simulink model "GUAM"  (R2023b)
settings: Solver=FixedStepAuto  StartTime=0.0  StopTime=SimIn.stopTime  FixedStep=Ts  RelTol=1e-3  AbsTol=1e-4  EnableMultiTasking=on
PostLoadFcn:
  | warning('off','sm:sli:setup:compile:LocalSolverNotSupported')
StartFcn:
  | tic
StopFcn:
  | Elapsed_Sim_Time = toc;
model workspace: external: MATLAB File aileronAssembly_DataFile.m (data not in the file)
values from neighbouring files (symbols this model uses):
  Ts = 0.05    [RUNME.m]
undefined symbols (not defined in the file or in its folder): AAC_Param, ang2Ext_coeff, Ki, Ki_scaling_elec, Kp, Leadscrew, motor_friction, R7_sctrl, sigbuilder_block, SimIn, SimPar, sm_aileron_actuator_lib, smiData, X, Y, Z
libraries: sm_lib x608, fl_lib x378, ee_lib x105, nesl_utility x96, simulink x10, eeGeneralControl x7, sh_lib x7, dspstat3 x6, sdl_lib x3, slpidlib x2, aerolibfltsims x2
(part 1 of 22)
Description:
  | Aileron Actuation System
  | 
  | Copyright 2018-2022 The MathWorks, Inc.
settings Model: NumberOfSteps=4  PacingRate=0.100000  Creator=smiller  LastModifiedBy=mkhaleghi
settings SolverCC: ConcurrentTasks=on  PositivePriorityOrder=on  AutoInsertRateTranBlk=on  InsertRTBMode=Never (minimum delay)
settings DataIOCC: MaxDataPoints=15000  SaveFormat=StructureWithTime  ReturnWorkspaceOutputs=off  SignalLoggingName=logsout_sm_aileron_actuator
settings OptimizationCC: BlockReduction=off  OptimizeBlockIOStorage=off  BufferReuse=off  ReuseModelBlockBuffer=off  GlobalBufferReuse=off  ExpressionFolding=off  LocalBlockOutputs=off  ZeroExternalMemoryAtStartup=off  ZeroInternalMemoryAtStartup=off  OptimizeDataStoreBuffers=off  BusAssignmentInplaceUpdate=off
settings DebuggingCC: UnconnectedInputMsg=warning  UnconnectedOutputMsg=warning  UnconnectedLineMsg=warning  PregeneratedLibrarySubsystemCodeDiagnostic=none  ArithmeticOperatorsInVariantConditions=warning
settings ModelReferenceCC: EnableRefExpFcnMdlSchedulingChecks=on
settings SFSimCC: SimUseLocalCustomCode=off  CustomCodeUndefinedFunction=UseInterfaceOnly
settings RTWCC: RTWUseLocalCustomCode=off  Toolchain=Simulink Real-Time Toolchain  BuildConfiguration=Faster Runs  TargetLang=C++  DLArmComputeVersion=19.05
settings GRTTargetCC: TargetLangStandard=C++03 (ISO)  CodeInterfacePackaging=C++ class
settings SimscapeCC: SimscapeLogType=all  SimscapeLogSimulationStatistics=on  SimscapeLogName=simlog_sm_aileron_actuator  SimscapeLogDataHistory=15000
settings DiagnosticsConfigSet: SimMechanicsJointTargetOverSpecification=none
settings ExplorerConfigSet: InternalSimMechanicsExplorerSettings="<ExplorerConfiguration><canonicalview>default</canonicalview><AnimationSetting><BasePlaybackSpeed>1.0</BasePlaybackSpeed><PlaybackSpeedFactor>1.0</PlaybackSpeedFactor></AnimationSetting><TilePanel><TileInfo><Tiles Columns=\"1\" Count=\"2\" Rows=\"2\"><Column Weight=\"1\"/><Row Weight=\"0.4705\"/><Row Weight=\"0.5295\"/><Tile Height=\"1\" Width=\"1\" X=\"0\" Y=\"0\"/><Tile Height=\"1\" Width=\"1\" X=\"0\" Y=\"1\"/></Tiles></TileInfo><SceneInfo><SceneViewer><BGColor><R>1</R><G>1</G><B>1</B></BGColor><Camera><DoPerspective>off</DoPerspective><Position><X>1.23761627695084986</X><Y>-8.90758678936009929</Y><Z>1.00676905686621598</Z></Position><Center><X>1.32324875041682244</X><Y>-5.82226757680397977</Y><Z>0.958078552790263771</Z></Center><Up><X>0.0220880463597219329</X><Y>0.0151626360058847443</Y><Z>0.999641041913228001</Z></Up><ViewLimDist>1</ViewLimDist><YLim>0.212915807710631483</YLim><XLim>0.504029784798622149</XLim></Camera></SceneViewer><SceneViewer><BGColor><R>1</R><G>1</G><B>1</B></BGColor><Camera><DoPerspective>off</DoPerspective><Position><X>0.794396209708300383</X><Y>-9.38995557415099746</Y><Z>3.30429825173386327</Z></Position><Center><X>1.22507763881924903</X><Y>-6.96050137175265426</Y><Z>-0.946177962255213334</Z></Center><Up><X>0.0136714074370919147</X><Y>0.867510835818079196</Y><Z>0.497230371514961633</Z></Up><ViewLimDist>1</ViewLimDist><YLim>0.0698383925509900721</YLim><XLim>0.146660624357079161</XLim></Camera></SceneViewer></SceneInfo></TilePanel><MechEditorPanel><Cameras/><GfxPanelCameraMap/><VideoCreator><PlaybackSpeedRatio>1.0</PlaybackSpeedRatio><FrameRate>30</FrameRate><VideoFormat>Motion JPEG AVI</VideoFormat><FrameSize>auto</FrameSize></VideoCreator></MechEditorPanel></ExplorerConfiguration>"

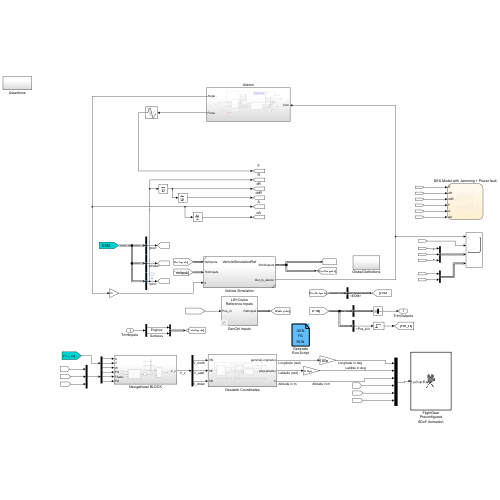
[thumbnail: Simulink's stored preview of the top-level diagram]
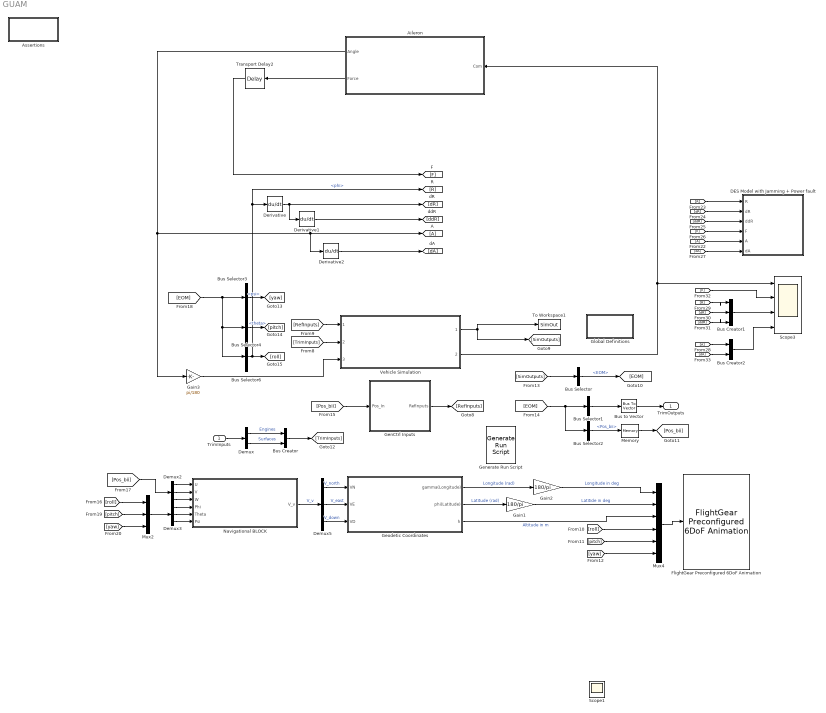
== system GUAM ==
  TrimInputs : Inport
  A : Goto
  Aileron : Subsystem
  Assertions : Subsystem
  Bus Creator : BusCreator  Inputs=2  OutDataTypeStr=Bus: BUS_TRIM_INPUT
  Bus Creator1 : BusCreator  Inputs=3
  Bus Creator2 : BusCreator  Inputs=2
  Bus Selector : BusSelector  OutputSignals=Vehicle.EOM
  Bus Selector1 : BusSelector  OutputSignals=AirRelativeData.Veas,AirRelativeData.Vtot,AirRelativeData.alpha,AirRelativeData.beta,WorldRelativeData.gamma,WorldRelativeData.chi,InertialData.Asensed_bIb,AirRelativeData.Vtotdot,AirRelativeData.alphadot,AirRelativeData.betadot,WorldRelativeData.gammadot,WorldRelativeData.chidot,WorldRelativeData.VelDtH_bEh,WorldRelativeData.Euler.phi,WorldRelativeData.Euler.theta,WorldRelativeData.Euler.psi  OutputAsBus=on
  Bus Selector2 : BusSelector  OutputSignals=InertialData.Pos_bii
  Bus Selector3 : BusSelector  OutputSignals=WorldRelativeData.Euler.psi
  Bus Selector4 : BusSelector  OutputSignals=WorldRelativeData.Euler.theta
  Bus Selector6 : BusSelector  OutputSignals=WorldRelativeData.Euler.phi
  Bus to Vector : BusToVector
  DES Model with Jamming + Power fault : Stateflow chart  TreatAsAtomicUnit=on
      settings: PortSchema="{\"entries\":[{\"content\":{\"sides\":[{\"content\":{},\"type\":\"ConnectorPlacement.EquallySpacedRectSide\",\"uuid\":\"a67ccfb6-3a22-4184-959b-082339053208\"},{\"content\":{\"side\":\"RIGHT\"},\"type\":\"ConnectorPlacement.EquallySpacedRectSide\",\"uuid\":\"6d92a68e-2e9e-4c9c-ac97-2465a38c08e0\"},{\"content\":{\"side\":\"TOP\"},\"type\":\"ConnectorPlacement.EquallySpacedRectSide\",\"uuid\":\"ae8db2dd-ba89-4797-9154-20cef1450f5e\"},{\"content\":{\"connectorIds\":[\"In1\",\"In2\",\"In5\",\"In4\",\"In3\",\"In6\"],\"side\":\"BOTTOM\"},\"type\":\"ConnectorPlacement.EquallySpacedRectSide\",\"uuid\":\"4d772bfb-b5db-457d-b647-bdd980a0fe5b\"}]},\"type\":\"ConnectorPlacement.EquallySpacedConnector\",\"uuid\":\"6e87b71b-43ed-4efe-bae7-cb7d2639d285\"}],\"packageUris\":[\"http://schema.mathworks.com/mf0/Connector/R2020b\"],\"version\":\"1.0\"}"
  Demux : Demux  Outputs=[SimIn.Trim.numEngines SimIn.Trim.numSurfaces]
  Demux2 : Demux  Outputs=3
  Demux3 : Demux  Outputs=3
  Demux5 : Demux  Outputs=3
  Derivative : Derivative
  Derivative1 : Derivative
  Derivative2 : Derivative
  FlightGear Preconfigured 6DoF Animation : aerolibfltsims/FlightGear Preconfigured 6DoF Animation  xFlightGearVersion=v2019.1  DestinationIpAddress=127.0.0.1  DestinationPort=5502  SampleTime=Ts  packetVersion=24
  From22 : From
  From28 : From
  Gain1 : Gain  Gain=180/pi
  Gain2 : Gain  Gain=180/pi
  Gain3 : Gain  Gain=pi/180
  GenCtrl Inputs : Subsystem  Variant=on  VariantControl=Variant1
  Generate Run Script : aerolibfltsims/Generate Run Script  Architecture=Win64  dataFlow=Send  GeometryModelName=c172p  AirportId=KJFK  RunwayId=13L  InitialAltitude=1100  InitialHeading=113  OffsetDistance=0  OffsetAzimuth=0  InstallScenery=off  DisableShaders=on  OriginAddress=127.0.0.1  DestinationPort=5502  OriginPort=5505  LocalAddress=127.0.0.1  OutputFileName=runfg.bat  FlightGearBaseDirectory=C:\Program Files\FlightGear 2020.3
  Geodetic Coordinates : Subsystem
  Global Definitions : Subsystem
  Memory : Memory
  Mux2 : Mux  Inputs=3
  Mux4 : Mux  Inputs=6
  Navigational BLOCK : Subsystem
  Scope3 : Scope  NumInputPorts=4
  To Workspace1 : ToWorkspace  VariableName=SimOut  SaveFormat=Timeseries  SampleTime=-1
      settings: Save2DSignal=2-D array (concatenate along first dimension)
  Transport Delay2 : TransportDelay  DelayTime=0.3
  Vehicle Simulation : Subsystem  ReferencedSubsystem=VehicleSimulationRef
  TrimOutputs : Outport  OutDataTypeStr=double  VectorParamsAs1DForOutWhenUnconnected=off
  Scope1 : Scope
  wires:
  Bus Selector4/1 -> [pitch]  "<theta>"
  [pitch] -> Mux4/5
  [pitch] -> Mux2/2
  Demux3/3 -> Navigational BLOCK/6(Psi)
  Gain1/1 -> Mux4/2  "Latitide in deg"
  [Pos_bii] -> GenCtrl Inputs/1(Pos_In)
  Mux2/1 -> Demux3/1
  Demux3/2 -> Navigational BLOCK/5(Theta)
  Geodetic Coordinates/3(h) -> Mux4/3  "Altitude in m"
  Geodetic Coordinates/1(gamma(Longitude)) -> Gain2/1  "Longitude (rad)"
  Bus Selector3/1 -> [yaw]  "<psi>"
  Bus Selector1/1 -> Bus to Vector/1
  Demux5/1 -> Geodetic Coordinates/1(VN)  "V_north"
  Demux5/3 -> Geodetic Coordinates/3(VD)  "V_down"
  Geodetic Coordinates/2(phi(Latitude)) -> Gain1/1  "Latitude (rad)"
  Demux2/2 -> Navigational BLOCK/2(V)
  [EOM] -> Bus Selector6/1, Bus Selector4/1, Bus Selector3/1
  [yaw] -> Mux2/3
  Navigational BLOCK/1(V_v) -> Demux5/1  "V_v"
  Demux2/1 -> Navigational BLOCK/1(U)
  [EOM] -> Bus Selector1/1, Bus Selector2/1
  Demux3/1 -> Navigational BLOCK/4(Phi)
  Bus Selector/1 -> [EOM]  "<EOM>"
  Memory/1 -> [Pos_bii]
  Demux2/3 -> Navigational BLOCK/3(W)
  GenCtrl Inputs/1(RefInputs) -> [RefInputs]
  [roll] -> Mux4/4
  Bus Selector2/1 -> Memory/1  "<Pos_bii>"
  Demux5/2 -> Geodetic Coordinates/2(VE)  "V_east"
  [RefInputs] -> Vehicle Simulation/1
  [yaw] -> Mux4/6
  Vehicle Simulation/1 -> To Workspace1/1, [SimOutputs]
  [roll] -> Mux2/1
  [TrimInputs] -> Vehicle Simulation/2
  Demux/1 -> Bus Creator/1  "Engines"
  [SimOutputs] -> Bus Selector/1
  TrimInputs/1 -> Demux/1
  Mux4/1 -> FlightGear Preconfigured 6DoF Animation/1
  Bus to Vector/1 -> TrimOutputs/1
  Bus Selector6/1 -> [roll], [R], Derivative/1  "<phi>"
  Gain2/1 -> Mux4/1  "Longitude in deg"
  Bus Creator/1 -> [TrimInputs]
  [Pos_bii] -> Demux2/1
  Demux/2 -> Bus Creator/2  "Surfaces"
  Gain3/1 -> Vehicle Simulation/3
  Vehicle Simulation/2 -> Scope3/1, Aileron/1(Com)
  Derivative/1 -> [dR], Derivative1/1
  Derivative1/1 -> [ddR]
  Aileron/1(Angle) -> Gain3/1, Derivative2/1, A/1
  Aileron/2(Force) -> Transport Delay2/1
  Transport Delay2/1 -> [F]
  Derivative2/1 -> [dA]
  [R] -> DES Model with Jamming + Power fault/1(R)
  [dR] -> DES Model with Jamming + Power fault/2(dR)
  [ddR] -> DES Model with Jamming + Power fault/5(ddR)
  [F] -> DES Model with Jamming + Power fault/4(F)
  From22/1 -> DES Model with Jamming + Power fault/3(A)
  [dA] -> DES Model with Jamming + Power fault/6(dA)
  [F] -> Scope3/2
  [R] -> Bus Creator1/1
  [dR] -> Bus Creator1/2
  [ddR] -> Bus Creator1/3
  Bus Creator1/1 -> Scope3/3
  From28/1 -> Bus Creator2/1
  [dA] -> Bus Creator2/2
  Bus Creator2/1 -> Scope3/4

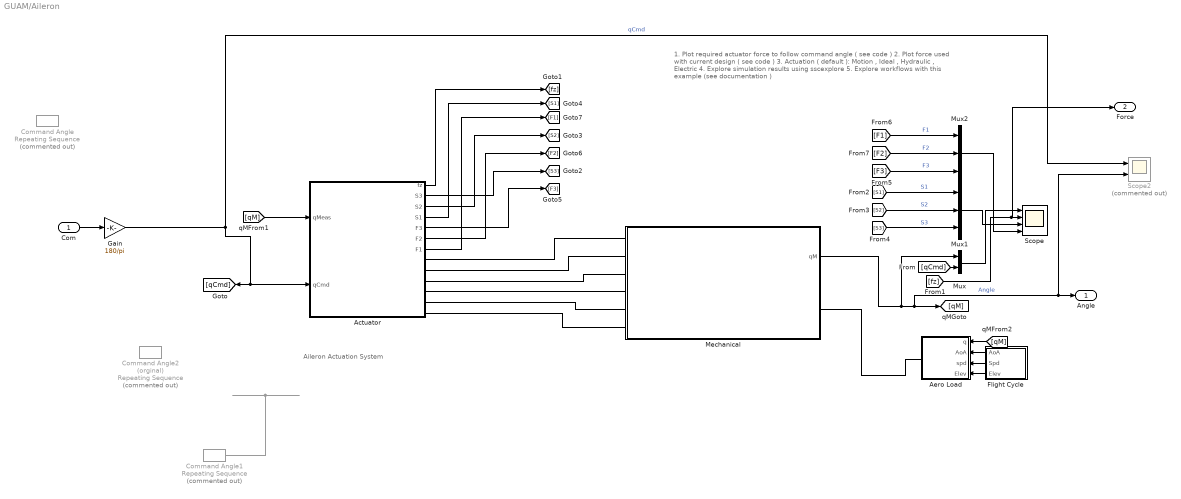
== system GUAM/Aileron ==
  note: 1. Plot required actuator force to follow command angle ( see code )
      | 2. Plot force used with current design ( see code )
      | 3. Actuation ( default ): Motion , Ideal , Hydraulic , Electric
      | 4. Explore simulation results using sscexplore
      | 5. Explore workflows with this example (see documentation )
  note: Aileron Actuation System
  Com : Inport
  Actuator : Subsystem  Tag=PublishSubsystem  Variant=on  VariantControlMode=label  VariantControl=Variant1  LabelModeActiveChoice=Electric
      settings: AttributesFormatString=%<ActiveVariant>
      mask Display:
      | Act_Char = get_param([bdroot '/Actuator'],'ActiveVariant');
      | SnC_Char = 'X';
      | PWM_Char = 'X';
      | if(strcmp(Act_Char(1),'E'))
      |     SnC_Char = get_param([bdroot '/Actuator/Electric/Leadscrew 1'],'popup_ctrl');
      |     PWM_Char = get_param([bdroot '/Actuator/Electric/Leadscrew 1'],'popup_driver');
      | end
      | 
      | image_str = ['sm_aileron_actuator_' Act_Char(1) 'sc' upper(SnC_Char(1)) 'pw' PWM_Char(1) '_IMAGE.png'];
      | 
      | try
      |     image(image_str);
      | catch
      | 
      | end
  Aero Load : Subsystem
  Command Angle : simulink/Sources/Repeating Sequence  Commented=on  rep_seq_t="[0.0 0.5 1.0 1.5  2.0  2.5  3.0   3.5  4.0   4.5    5.0   5.5  6.0   6.5  7.0   7.5  8.0  8.5  9.0  9.5   10.0]"  rep_seq_y="[0.0  0.0  0.0  0.0 5.0  10.0  10.0  0.0  0.0  -9.0  -17.5  -17.5  -10.0  0.0  2.0  6.0 15.0 15.0 6.0 3.0 -2.0]"
  Command Angle1 : simulink/Sources/Repeating Sequence  Commented=on  rep_seq_t="[0.0 0.5 1.0 1.5  2.0  2.5  3.0   3.5  4.0   4.5    5.0   5.5  6.0   6.5  7.0   7.5  8.0  8.5  9.0  9.5   10.0 10.5 11.0 11.5 12.0 12.5 13.0]"  rep_seq_y=|
      | [0
      | 0
      | 0
      | 0
      | 5
      | 10
      | 10
      | 0
      | 0
      | -10
      | -10
      | -10
      | 0
      | 0
      | 0
      | 6
      | 15
      | 15
      | 6
      | 0
      | -5
      | -5
      | 0
      | 0
      | 5
      | 10
      | 10]
  Command Angle2 (orginal) : simulink/Sources/Repeating Sequence  Commented=on  rep_seq_t="[0.0 0.5 1.0 1.5  2.0  2.5  3.0   3.5  4.0   4.5    5.0   5.5  6.0   6.5  7.0   7.5  8.0  8.5  9.0  9.5   10.0 10.5 11.0 11.5 12.0 12.5 13.0]"  rep_seq_y="[0.0  0.0  0.0  0.0 5.0  10.0  10.0  0.0  0.0  -9.0  -17.5  -17.5  -10.0  0.0  2.0  6.0 15.0 15.0 6.0 3.0 -2.0 -2.0 0 3.0 5.0 6.0 6.0]"
  Flight Cycle : Subsystem  Tag=STV Subsys  LoadFcn=sigbuilder_block('load');  StartFcn=sigbuilder_block('start');  StopFcn=sigbuilder_block('stop');  ClipboardFcn=sigbuilder_block('clipboard');  mask(Sigbuilder block){tuvar=[0:10]}
      mask help: Simulink:masks:SigbuilderBlock_MD
      mask init:
      | if ~strcmp(get_param(bdroot(gcbh),'SimulationStatus'),'stopped') tuvar = sigbuilder_block('maskInit'); end
      settings: CopyFcn=sigbuilder_block('copy');  DeleteFcn=sigbuilder_block('delete');  ModelCloseFcn=sigbuilder_block('modelClose');  PreSaveFcn=sigbuilder_block('preSave');  PauseFcn=sigbuilder_block('pause');  ContinueFcn=sigbuilder_block('continue');  NameChangeFcn=sigbuilder_block('namechange');  OpenFcn=sigbuilder_block('open',[440.4 133.2 550.8 400.2 ]);  CloseFcn=sigbuilder_block('close');
      mask Display: plot(0, 0, 100, 100,[2, 2, 32, 32, 2], [68, 8, 8, 68, 68],[32, 2], [38, 38], [32, 19, 2],[53, 60, 44], [32, 17, 17, 2],[16, 16, 31, 31]);txt = getActiveGroup(gcbh);text(2, 100, txt,'verticalAlignment', 'top');
  Gain : Gain  Gain=180/pi
  Mechanical : Subsystem  Tag=PublishSubsystem
      mask Display: image('sm_aileron_actuator_aileron_full_IMAGE.png');
  Mux : Mux  Inputs=2
  Mux1 : Mux  Inputs=3
  Mux2 : Mux  Inputs=3
  Scope : Scope  NumInputPorts=4
  Scope2 : Scope  Commented=on  NumInputPorts=2
  Angle : Outport
  Force : Outport  Port=2
  wires:
  Command Angle1/1 -> ?
  Mux1/1 -> Scope/3
  Mux/1 -> Scope/1
  Mux2/1 -> Scope/4
  [F3] -> Mux2/3  "F3"
  Actuator/3(S2) -> [S2]
  Gain/1 -> Scope2/1, Actuator/2("qCmd "), [qCmd]  "qCmd"
  Actuator/4(S1) -> [S1]
  Actuator/6(F2) -> [F2]
  Flight Cycle/2(Spd) -> Aero Load/3(spd)
  Actuator/5(F3) -> [F3]
  [F2] -> Mux2/2  "F2"
  Actuator/7(F1) -> [F1]
  [qM] -> Aero Load/1(q)
  Flight Cycle/3(Elev) -> Aero Load/4(Elev)
  [qM] -> Actuator/1(qMeas)
  Actuator/2(S3) -> [S3]
  Mechanical/1(qM) -> Angle/1, Scope2/2, [qM], Mux/1  "Angle"
  [S1] -> Mux1/1  "S1"
  [fz] -> Force/1, Scope/2
  [S3] -> Mux1/3  "S3"
  [qCmd] -> Mux/2
  [F1] -> Mux2/1  "F1"
  Flight Cycle/1(AoA) -> Aero Load/2(AoA)
  Actuator/1(" fz") -> [fz]
  [S2] -> Mux1/2  "S2"
  Com/1 -> Gain/1
  connections:
  Actuator/RConn3 -- Mechanical/LConn3
  Actuator/RConn4 -- Mechanical/LConn4
  Actuator/RConn5 -- Mechanical/LConn5
  Aero Load/RConn1 -- Mechanical/RConn1
  Actuator/RConn6 -- Mechanical/LConn6
  Actuator/RConn1 -- Mechanical/LConn1
  Actuator/RConn2 -- Mechanical/LConn2

== system GUAM/Assertions ==
  Clock1 : Clock
  Compare To Constant : simulink/Logic and Bit Operations/Compare To Constant  relop=>=  const=0.2  OutDataTypeStr=boolean  ZeroCross=off
  Constant2 : Constant  Value=SimIn.Switches.TrimModeOn
  Constant3 : Constant  Value=SimIn.Switches.LinearizeModeOn
  KillifNotSimMode : Assertion  AssertionFailFcn="warndlg('Running simulation with TrimMode or LinearizeMode engaged.  Run setup.m to reset.','Warning!')"
  Logical Operator : Logic  Operator=NAND  AllPortsSameDT=off  OutDataTypeStr=boolean
  Logical Operator1 : Logic  Operator=OR  AllPortsSameDT=off  OutDataTypeStr=boolean
  wires:
  Constant2/1 -> Logical Operator1/1
  Compare To Constant/1 -> Logical Operator/2
  Clock1/1 -> Compare To Constant/1
  Logical Operator/1 -> KillifNotSimMode/1
  Constant3/1 -> Logical Operator1/2
  Logical Operator1/1 -> Logical Operator/1

== system GUAM/GenCtrl Inputs ==
  Pos_In : Inport
  GL-10 Reference Inputs : Subsystem  VariantControl=GVS_VEH_TYPE_GL10  ReferencedSubsystem=GL_10_Reference_Inputs
  Generic Tilt Rotor Reference Inputs : Subsystem  VariantControl=GVS_VEH_TYPE_GTR  ReferencedSubsystem=GTR_Reference_Inputs
  Generic Tilt Wing Reference Inputs : Subsystem  VariantControl=GVS_VEH_TYPE_GTW  ReferencedSubsystem=GTW_Reference_Inputs
  LA-8 Reference Inputs : Subsystem  VariantControl=GVS_VEH_TYPE_LA8  ReferencedSubsystem=LA_8_Reference_Inputs
  Lift+Cruise Reference Inputs : Subsystem  VariantControl=GVS_VEH_TYPE_LC  ReferencedSubsystem=Lift_Cruise_Reference_Inputs
  Quad6 Reference Inputs : Subsystem  VariantControl=GVS_VEH_TYPE_QUAD6  ReferencedSubsystem=Quad6_Reference_Inputs
  RefInputs : Outport  OutDataTypeStr=Bus: BUS_REF_INPUT

== system GUAM/Geodetic Coordinates ==
  VN : Inport
  VE : Inport  Port=2
  VD : Inport  Port=3
  Gain : Gain  Gain=-1
  Integrator : Integrator  InitialCondition=150
  Integrator1 : Integrator  InitialCondition=0.22181
  Integrator2 : Integrator  InitialCondition=1.356068
  LATITUDE : MATLAB Function  TreatAsAtomicUnit=on
  LONGITUDE : MATLAB Function  TreatAsAtomicUnit=on
  M and N : Subsystem
  gamma(Longitude) : Outport
  phi(Latitude) : Outport  Port=2
  h : Outport  Port=3
  wires:
  VD/1 -> Gain/1  "VD"
  Gain/1 -> Integrator/1  "h_dot"
  Integrator/1 -> LATITUDE/3(h), LONGITUDE/3(h), h/1  "h"
  M and N/1(M) -> LATITUDE/2(M)
  M and N/2(N) -> LONGITUDE/2(N)
  LATITUDE/1(phi_dot) -> Integrator1/1  "phi_dot"
  Integrator1/1 -> LONGITUDE/4(phi), M and N/1(phi), phi(Latitude)/1  "phi"
  VE/1 -> LONGITUDE/1(VE)  "VE"
  VN/1 -> LATITUDE/1(VN)  "VN"
  LONGITUDE/1(gamma_dot) -> Integrator2/1  "gamma_dot"
  Integrator2/1 -> gamma(Longitude)/1  "gamma"

== system GUAM/Global Definitions ==
  EOM_IC : Constant  Value=SimPar.EOM  OutDataTypeStr=Bus: BUS_PARAM_EOM
  IC : Constant  Value=SimPar.IC  OutDataTypeStr=Bus: BUS_PARAM_IC
  Terminator : Terminator
  Terminator1 : Terminator
  tag scope: EOM_IC=global, IC=global
  wires:
  IC/1 -> [IC]
  EOM_IC/1 -> [EOM_IC]
  [IC] -> Terminator/1
  [EOM_IC] -> Terminator1/1

== system GUAM/Navigational BLOCK ==
  U : Inport
  V : Inport  Port=2
  W : Inport  Port=3
  Phi : Inport  Port=4
  Theta : Inport  Port=5
  Psi : Inport  Port=6
  Math Function : Math  Operator=transpose
  Matrix Multiply : Product  Multiplication=Matrix(*)
  Mux2 : Mux  Inputs=3
  Navigational Equation : Subsystem
  V_v : Outport
  wires:
  V/1 -> Mux2/2
  Psi/1 -> Navigational Equation/3(phi)
  W/1 -> Mux2/3
  Navigational Equation/1(C_B/V) -> Math Function/1
  Matrix Multiply/1 -> V_v/1
  Theta/1 -> Navigational Equation/2(theat)
  U/1 -> Mux2/1
  Phi/1 -> Navigational Equation/1(psi)
  Math Function/1 -> Matrix Multiply/1
  Mux2/1 -> Matrix Multiply/2

== system GUAM/Aileron/Actuator ==
  qMeas : Inport
  "qCmd " : Inport  Port=2
  Electric : Subsystem  VariantControl=Electric
      mask Display: image('sm_aileron_actuator_EscXpwX_IMAGE.png');
  Hydraulic : Subsystem  VariantControl=Hydraulic
      mask Display: image('sm_aileron_actuator_HscXpwX_IMAGE.png');
  Ideal : Subsystem  VariantControl=Ideal
      mask Display: image('sm_aileron_actuator_IscXpwX_IMAGE.png');
  Motion : Subsystem  VariantControl=Motion
      mask Display: image('sm_aileron_actuator_MscXpwX_IMAGE.png');
  " C1" : PMIOPort  Side=Right
  " P1" : PMIOPort  Port=2  Side=Right
  " C2" : PMIOPort  Port=3  Side=Right
  " P2" : PMIOPort  Port=4  Side=Right
  " C3" : PMIOPort  Port=5  Side=Right
  " P3" : PMIOPort  Port=6  Side=Right
  " fz" : Outport  VectorParamsAs1DForOutWhenUnconnected=off
  S3 : Outport  Port=2
  S2 : Outport  Port=3
  S1 : Outport  Port=4
  F3 : Outport  Port=5
  F2 : Outport  Port=6
  F1 : Outport  Port=7

== system GUAM/Aileron/Aero Load ==
  note: Proof of concept calculation only.
      | Realistic values must be obtained from literature or experimentation.
  q : Inport
  AoA : Inport  Port=2
  spd : Inport  Port=3
  Elev : Inport  Port=4
  Aerodynamic Hinge Moment : sm_lib/Forces and Torques/External Force and Torque  ForceResolutionFrame=AttachedFrame  EnableForceX=off  EnableForceY=off  EnableForceZ=off  EnableForce=off  TorqueResolutionFrame=AttachedFrame  EnableTorqueX=off  EnableTorqueY=on  EnableTorqueZ=off  EnableTorque=off
  Gain : Gain  Gain=0.5
  Math Function : Math  Operator=square  SignedPower=on
  Product : Product  Inputs=4
  Scaling : Gain  Gain=1e-6
  Simulink-PS Converter : nesl_utility/Simulink-PS Converter  PhysicalDomain=network_engine_domain  SubClassName=ps_input  LeftPortType=input  RightPortType=output  PseudoPeriodic=off  Frequencies=[]  NoiseDistribution=none  NoiseParameters=[]  Unit=1  AffineConversion=off  FilteringAndDerivatives=provide  SimscapeFilterOrder=1  InputFilterTimeConstant=0.005  UdotUserProvided=0
  Table AoA : Lookup_n-D  NumberOfTableDimensions=1  BreakpointsForDimension1=[-5:5]  Table=tanh([-5:5])  InternalRulePriority=Speed  RndMeth=Simplest
  Table Elev : Lookup_n-D  NumberOfTableDimensions=1  BreakpointsForDimension1=[-5:5]  Table=tanh([-5:5])  InternalRulePriority=Speed  RndMeth=Simplest
  Table q : Lookup_n-D  NumberOfTableDimensions=1  BreakpointsForDimension1=[-5:5]  Table=tanh([-5:5])  InternalRulePriority=Speed  RndMeth=Simplest
  A : PMIOPort  Side=Right
  wires:
  Gain/1 -> Scaling/1
  AoA/1 -> Table AoA/1
  q/1 -> Table q/1
  spd/1 -> Math Function/1
  Elev/1 -> Table Elev/1
  Table q/1 -> Product/1
  Table AoA/1 -> Product/2
  Math Function/1 -> Product/3
  Table Elev/1 -> Product/4  "rho"
  Product/1 -> Gain/1
  Scaling/1 -> Simulink-PS Converter/1
  connections:
  Simulink-PS Converter/RConn1 -- Aerodynamic Hinge Moment/LConn1
  Aerodynamic Hinge Moment/RConn1 -- A/RConn1

== system GUAM/Aileron/Flight Cycle ==
  Demux : Demux  Tag=STV Demux  Outputs=3
      settings: DisplayOption=none
  FromWs : FromWorkspace  Tag=STV FromWs  VariableName=tuvar
      SigBuilderData=|
      | common.afterFinalStr = 'Extrapolate'
      | common.sampleTime = 0
      | dataSet.timeRange = [0 10]
      | dataSet.name = 'FC1'
      | sbobj.Groups.Name = 'FC1'
      | sbobj.Groups.Signals(1).Name = 'AoA'
      | sbobj.Groups.Signals(1).XData = [0 10]
      | sbobj.Groups.Signals(1).YData = [1 1]
      | sbobj.Groups.Signals(2).Name = 'Spd'
      | sbobj.Groups.Signals(2).XData = [0 10]
      | sbobj.Groups.Signals(2).YData = [1000 1000]
      | sbobj.Groups.Signals(3).Name = 'Elev'
      | sbobj.Groups.Signals(3).XData = [0 10]
      | sbobj.Groups.Signals(3).YData = [300 300]
  AoA : Outport  Tag=STV Outport  VectorParamsAs1DForOutWhenUnconnected=off
  Spd : Outport  Tag=STV Outport  Port=2  VectorParamsAs1DForOutWhenUnconnected=off
  Elev : Outport  Tag=STV Outport  Port=3  VectorParamsAs1DForOutWhenUnconnected=off
  wires:
  Demux/1 -> AoA/1
  FromWs/1 -> Demux/1
  Demux/2 -> Spd/1
  Demux/3 -> Elev/1

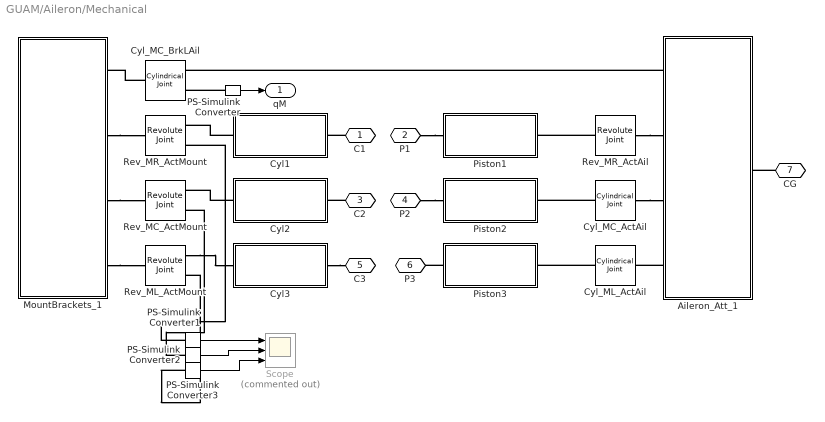
== system GUAM/Aileron/Mechanical ==
  Aileron_Att_1 : Subsystem  Tag=PublishSubsystem
      mask Display: image('sm_aileron_actuator_aileron_assy_IMAGE.png');
  Cyl1 : Subsystem
      mask Display: image('sm_aileron_actuator_aileron_cylinder_IMAGE.png');
  Cyl2 : Subsystem
      mask Display: image('sm_aileron_actuator_aileron_cylinder_IMAGE.png');
  Cyl3 : Subsystem
      mask Display: image('sm_aileron_actuator_aileron_cylinder_IMAGE.png');
  Cyl_MC_ActAil : sm_lib/Joints/Cylindrical Joint  JointMode=Normal  SenseConstraintForce=off  SenseConstraintForceX=off  SenseConstraintForceY=off  SenseConstraintForceZ=off  SenseConstraintTorque=off  SenseConstraintTorqueX=off  SenseConstraintTorqueY=off  SenseConstraintTorqueZ=off  SenseTotalForce=off  SenseTotalForceX=off  SenseTotalForceY=off  SenseTotalForceZ=off  SenseTotalTorque=off  SenseTotalTorqueX=off  SenseTotalTorqueY=off  SenseTotalTorqueZ=off  CompositeWrenchDir=FollowerOnBase  CompositeWrenchFrame=BaseFrame  PzEquilibriumPosition=0  PzEquilibriumPositionUnits=m  PzSpringStiffness=0  PzSpringStiffnessUnits=N/m  PzDampingCoefficient=0  PzDampingCoefficientUnits=N/(m/s)  PzTorqueActuationMode=NoTorque  PzMotionActuationMode=ComputedMotion  PzSensePosition=off  PzSenseVelocity=off  PzSenseAcceleration=off  PzSenseTorqueForce=off  PzSenseLowerLimitTorqueForce=off  PzSenseUpperLimitTorqueForce=off  PzLowerLimitSpecify=off  PzLowerLimitBound=-1  PzLowerLimitBoundUnits=m  PzLowerLimitStiffness=1e6  PzLowerLimitStiffnessUnits=N/m  PzLowerLimitDamping=1e3  PzLowerLimitDampingUnits=N/(m/s)  PzLowerLimitTransitionRegionWidth=1e-4  PzLowerLimitTransitionRegionWidthUnits=m  PzUpperLimitSpecify=off  PzUpperLimitBound=1  PzUpperLimitBoundUnits=m  PzUpperLimitStiffness=1e6  PzUpperLimitStiffnessUnits=N/m  PzUpperLimitDamping=1e3  PzUpperLimitDampingUnits=N/(m/s)  PzUpperLimitTransitionRegionWidth=1e-4  PzUpperLimitTransitionRegionWidthUnits=m  PzPositionTargetSpecify=on  PzPositionTargetPriority=Low  PzPositionTargetValue=smiData.CylindricalJoint(5).Pz.Pos  PzPositionTargetValueUnits=m  PzVelocityTargetSpecify=off  PzVelocityTargetPriority=High  PzVelocityTargetValue=0  PzVelocityTargetValueUnits=m/s  RzEquilibriumPosition=0  RzEquilibriumPositionUnits=rad  RzSpringStiffness=0  RzSpringStiffnessUnits=N*m/rad  RzDampingCoefficient=0  RzDampingCoefficientUnits=N*m/(rad/s)  RzTorqueActuationMode=NoTorque  RzMotionActuationMode=ComputedMotion  RzSensePosition=off  RzSenseVelocity=off  RzSenseAcceleration=off  RzSenseTorqueForce=off  RzSenseLowerLimitTorqueForce=off  RzSenseUpperLimitTorqueForce=off  RzLowerLimitSpecify=off  RzLowerLimitBound=-90  RzLowerLimitBoundUnits=deg  RzLowerLimitStiffness=1e4  RzLowerLimitStiffnessUnits=N*m/deg  RzLowerLimitDamping=10  RzLowerLimitDampingUnits=N*m/(deg/s)  RzLowerLimitTransitionRegionWidth=0.1  RzLowerLimitTransitionRegionWidthUnits=deg  RzUpperLimitSpecify=off  RzUpperLimitBound=90  RzUpperLimitBoundUnits=deg  RzUpperLimitStiffness=1e4  RzUpperLimitStiffnessUnits=N*m/deg  RzUpperLimitDamping=10  RzUpperLimitDampingUnits=N*m/(deg/s)  RzUpperLimitTransitionRegionWidth=0.1  RzUpperLimitTransitionRegionWidthUnits=deg  RzPositionTargetSpecify=on  RzPositionTargetPriority=Low  RzPositionTargetValue=smiData.CylindricalJoint(5).Rz.Pos  RzPositionTargetValueUnits=deg  RzVelocityTargetSpecify=off  RzVelocityTargetPriority=High  RzVelocityTargetValue=0  RzVelocityTargetValueUnits=deg/s
  Cyl_MC_BrkLAil : sm_lib/Joints/Cylindrical Joint  JointMode=Normal  SenseConstraintForce=off  SenseConstraintForceX=off  SenseConstraintForceY=off  SenseConstraintForceZ=off  SenseConstraintTorque=off  SenseConstraintTorqueX=off  SenseConstraintTorqueY=off  SenseConstraintTorqueZ=off  SenseTotalForce=off  SenseTotalForceX=off  SenseTotalForceY=off  SenseTotalForceZ=off  SenseTotalTorque=off  SenseTotalTorqueX=off  SenseTotalTorqueY=off  SenseTotalTorqueZ=off  CompositeWrenchDir=FollowerOnBase  CompositeWrenchFrame=BaseFrame  PzEquilibriumPosition=0  PzEquilibriumPositionUnits=m  PzSpringStiffness=0  PzSpringStiffnessUnits=N/m  PzDampingCoefficient=0  PzDampingCoefficientUnits=N/(m/s)  PzTorqueActuationMode=NoTorque  PzMotionActuationMode=ComputedMotion  PzSensePosition=off  PzSenseVelocity=off  PzSenseAcceleration=off  PzSenseTorqueForce=off  PzSenseLowerLimitTorqueForce=off  PzSenseUpperLimitTorqueForce=off  PzLowerLimitSpecify=off  PzLowerLimitBound=-1  PzLowerLimitBoundUnits=m  PzLowerLimitStiffness=1e6  PzLowerLimitStiffnessUnits=N/m  PzLowerLimitDamping=1e3  PzLowerLimitDampingUnits=N/(m/s)  PzLowerLimitTransitionRegionWidth=1e-4  PzLowerLimitTransitionRegionWidthUnits=m  PzUpperLimitSpecify=off  PzUpperLimitBound=1  PzUpperLimitBoundUnits=m  PzUpperLimitStiffness=1e6  PzUpperLimitStiffnessUnits=N/m  PzUpperLimitDamping=1e3  PzUpperLimitDampingUnits=N/(m/s)  PzUpperLimitTransitionRegionWidth=1e-4  PzUpperLimitTransitionRegionWidthUnits=m  PzPositionTargetSpecify=on  PzPositionTargetPriority=Low  PzPositionTargetValue=smiData.CylindricalJoint(4).Pz.Pos  PzPositionTargetValueUnits=m  PzVelocityTargetSpecify=off  PzVelocityTargetPriority=High  PzVelocityTargetValue=0  PzVelocityTargetValueUnits=m/s  RzEquilibriumPosition=0  RzEquilibriumPositionUnits=rad  RzSpringStiffness=0  RzSpringStiffnessUnits=N*m/rad  RzDampingCoefficient=0  RzDampingCoefficientUnits=N*m/(rad/s)  RzTorqueActuationMode=NoTorque  RzMotionActuationMode=ComputedMotion  RzSensePosition=on  RzSenseVelocity=off  RzSenseAcceleration=off  RzSenseTorqueForce=off  RzSenseLowerLimitTorqueForce=off  RzSenseUpperLimitTorqueForce=off  RzLowerLimitSpecify=off  RzLowerLimitBound=-90  RzLowerLimitBoundUnits=deg  RzLowerLimitStiffness=1e4  RzLowerLimitStiffnessUnits=N*m/deg  RzLowerLimitDamping=10  RzLowerLimitDampingUnits=N*m/(deg/s)  RzLowerLimitTransitionRegionWidth=0.1  RzLowerLimitTransitionRegionWidthUnits=deg  RzUpperLimitSpecify=off  RzUpperLimitBound=90  RzUpperLimitBoundUnits=deg  RzUpperLimitStiffness=1e4  RzUpperLimitStiffnessUnits=N*m/deg  RzUpperLimitDamping=10  RzUpperLimitDampingUnits=N*m/(deg/s)  RzUpperLimitTransitionRegionWidth=0.1  RzUpperLimitTransitionRegionWidthUnits=deg  RzPositionTargetSpecify=on  RzPositionTargetPriority=Low  RzPositionTargetValue=smiData.CylindricalJoint(4).Rz.Pos  RzPositionTargetValueUnits=deg  RzVelocityTargetSpecify=off  RzVelocityTargetPriority=High  RzVelocityTargetValue=0  RzVelocityTargetValueUnits=deg/s
  Cyl_ML_ActAil : sm_lib/Joints/Cylindrical Joint  JointMode=Normal  SenseConstraintForce=off  SenseConstraintForceX=off  SenseConstraintForceY=off  SenseConstraintForceZ=off  SenseConstraintTorque=off  SenseConstraintTorqueX=off  SenseConstraintTorqueY=off  SenseConstraintTorqueZ=off  SenseTotalForce=off  SenseTotalForceX=off  SenseTotalForceY=off  SenseTotalForceZ=off  SenseTotalTorque=off  SenseTotalTorqueX=off  SenseTotalTorqueY=off  SenseTotalTorqueZ=off  CompositeWrenchDir=FollowerOnBase  CompositeWrenchFrame=BaseFrame  PzEquilibriumPosition=0  PzEquilibriumPositionUnits=m  PzSpringStiffness=0  PzSpringStiffnessUnits=N/m  PzDampingCoefficient=0  PzDampingCoefficientUnits=N/(m/s)  PzTorqueActuationMode=NoTorque  PzMotionActuationMode=ComputedMotion  PzSensePosition=off  PzSenseVelocity=off  PzSenseAcceleration=off  PzSenseTorqueForce=off  PzSenseLowerLimitTorqueForce=off  PzSenseUpperLimitTorqueForce=off  PzLowerLimitSpecify=off  PzLowerLimitBound=-0.001  PzLowerLimitBoundUnits=m  PzLowerLimitStiffness=1e6  PzLowerLimitStiffnessUnits=N/m  PzLowerLimitDamping=1e3  PzLowerLimitDampingUnits=N/(m/s)  PzLowerLimitTransitionRegionWidth=1e-4  PzLowerLimitTransitionRegionWidthUnits=m  PzUpperLimitSpecify=off  PzUpperLimitBound=0.001  PzUpperLimitBoundUnits=m  PzUpperLimitStiffness=1e6  PzUpperLimitStiffnessUnits=N/m  PzUpperLimitDamping=1e3  PzUpperLimitDampingUnits=N/(m/s)  PzUpperLimitTransitionRegionWidth=1e-4  PzUpperLimitTransitionRegionWidthUnits=m  PzPositionTargetSpecify=on  PzPositionTargetPriority=Low  PzPositionTargetValue=smiData.CylindricalJoint(6).Pz.Pos  PzPositionTargetValueUnits=m  PzVelocityTargetSpecify=off  PzVelocityTargetPriority=High  PzVelocityTargetValue=0  PzVelocityTargetValueUnits=m/s  RzEquilibriumPosition=0  RzEquilibriumPositionUnits=rad  RzSpringStiffness=0  RzSpringStiffnessUnits=N*m/rad  RzDampingCoefficient=0  RzDampingCoefficientUnits=N*m/(rad/s)  RzTorqueActuationMode=NoTorque  RzMotionActuationMode=ComputedMotion  RzSensePosition=off  RzSenseVelocity=off  RzSenseAcceleration=off  RzSenseTorqueForce=off  RzSenseLowerLimitTorqueForce=off  RzSenseUpperLimitTorqueForce=off  RzLowerLimitSpecify=off  RzLowerLimitBound=-90  RzLowerLimitBoundUnits=deg  RzLowerLimitStiffness=1e4  RzLowerLimitStiffnessUnits=N*m/deg  RzLowerLimitDamping=10  RzLowerLimitDampingUnits=N*m/(deg/s)  RzLowerLimitTransitionRegionWidth=0.1  RzLowerLimitTransitionRegionWidthUnits=deg  RzUpperLimitSpecify=off  RzUpperLimitBound=90  RzUpperLimitBoundUnits=deg  RzUpperLimitStiffness=1e4  RzUpperLimitStiffnessUnits=N*m/deg  RzUpperLimitDamping=10  RzUpperLimitDampingUnits=N*m/(deg/s)  RzUpperLimitTransitionRegionWidth=0.1  RzUpperLimitTransitionRegionWidthUnits=deg  RzPositionTargetSpecify=on  RzPositionTargetPriority=Low  RzPositionTargetValue=smiData.CylindricalJoint(6).Rz.Pos  RzPositionTargetValueUnits=deg  RzVelocityTargetSpecify=off  RzVelocityTargetPriority=High  RzVelocityTargetValue=0  RzVelocityTargetValueUnits=deg/s
  MountBrackets_1 : Subsystem
      mask Display: image('sm_aileron_actuator_aileron_mounts_all_IMAGE.png');
  PS-Simulink Converter : nesl_utility/PS-Simulink Converter  PhysicalDomain=network_engine_domain  SubClassName=ps_output  LeftPortType=input  RightPortType=output  PseudoPeriodic=off  Frequencies=[]  VectorFormat=1-D array  Unit=deg  AffineConversion=off
  PS-Simulink Converter1 : nesl_utility/PS-Simulink Converter  PhysicalDomain=network_engine_domain  SubClassName=ps_output  LeftPortType=input  RightPortType=output  PseudoPeriodic=off  Frequencies=[]  VectorFormat=inherit  Unit=inherit  AffineConversion=off
  PS-Simulink Converter2 : nesl_utility/PS-Simulink Converter  PhysicalDomain=network_engine_domain  SubClassName=ps_output  LeftPortType=input  RightPortType=output  PseudoPeriodic=off  Frequencies=[]  VectorFormat=inherit  Unit=inherit  AffineConversion=off
  PS-Simulink Converter3 : nesl_utility/PS-Simulink Converter  PhysicalDomain=network_engine_domain  SubClassName=ps_output  LeftPortType=input  RightPortType=output  PseudoPeriodic=off  Frequencies=[]  VectorFormat=inherit  Unit=inherit  AffineConversion=off
  Piston1 : Subsystem
      mask Display: image('sm_aileron_actuator_aileron_piston_IMAGE.png');
  Piston2 : Subsystem
      mask Display: image('sm_aileron_actuator_aileron_piston_IMAGE.png');
  Piston3 : Subsystem
      mask Display: image('sm_aileron_actuator_aileron_piston_IMAGE.png');
  Rev_MC_ActMount : sm_lib/Joints/Revolute Joint  JointMode=Normal  SenseConstraintForce=off  SenseConstraintForceX=off  SenseConstraintForceY=off  SenseConstraintForceZ=off  SenseConstraintTorque=off  SenseConstraintTorqueX=off  SenseConstraintTorqueY=off  SenseConstraintTorqueZ=off  SenseTotalForce=off  SenseTotalForceX=off  SenseTotalForceY=off  SenseTotalForceZ=off  SenseTotalTorque=off  SenseTotalTorqueX=off  SenseTotalTorqueY=off  SenseTotalTorqueZ=off  CompositeWrenchDir=FollowerOnBase  CompositeWrenchFrame=BaseFrame  EquilibriumPosition=0  EquilibriumPositionUnits=rad  SpringStiffness=0  SpringStiffnessUnits=N*m/rad  DampingCoefficient=0  DampingCoefficientUnits=N*m/(rad/s)  TorqueActuationMode=NoTorque  MotionActuationMode=ComputedMotion  SensePosition=on  SenseVelocity=off  SenseAcceleration=off  SenseTorqueForce=off  SenseLowerLimitTorqueForce=off  SenseUpperLimitTorqueForce=off  LowerLimitSpecify=off  LowerLimitBound=-90  LowerLimitBoundUnits=deg  LowerLimitStiffness=1e4  LowerLimitStiffnessUnits=N*m/deg  LowerLimitDamping=10  LowerLimitDampingUnits=N*m/(deg/s)  LowerLimitTransitionRegionWidth=0.1  LowerLimitTransitionRegionWidthUnits=deg  UpperLimitSpecify=on  UpperLimitBound=90  UpperLimitBoundUnits=deg  UpperLimitStiffness=1e4  UpperLimitStiffnessUnits=N*m/deg  UpperLimitDamping=10  UpperLimitDampingUnits=N*m/(deg/s)  UpperLimitTransitionRegionWidth=0.1  UpperLimitTransitionRegionWidthUnits=deg  PositionTargetSpecify=on  PositionTargetPriority=Low  PositionTargetValue=smiData.RevoluteJoint(3).Rz.Pos  PositionTargetValueUnits=deg  VelocityTargetSpecify=off  VelocityTargetPriority=High  VelocityTargetValue=0  VelocityTargetValueUnits=deg/s
  Rev_ML_ActMount : sm_lib/Joints/Revolute Joint  JointMode=Normal  SenseConstraintForce=off  SenseConstraintForceX=off  SenseConstraintForceY=off  SenseConstraintForceZ=off  SenseConstraintTorque=off  SenseConstraintTorqueX=off  SenseConstraintTorqueY=off  SenseConstraintTorqueZ=off  SenseTotalForce=off  SenseTotalForceX=off  SenseTotalForceY=off  SenseTotalForceZ=off  SenseTotalTorque=off  SenseTotalTorqueX=off  SenseTotalTorqueY=off  SenseTotalTorqueZ=off  CompositeWrenchDir=FollowerOnBase  CompositeWrenchFrame=BaseFrame  EquilibriumPosition=0  EquilibriumPositionUnits=rad  SpringStiffness=0  SpringStiffnessUnits=N*m/rad  DampingCoefficient=0  DampingCoefficientUnits=N*m/(rad/s)  TorqueActuationMode=NoTorque  MotionActuationMode=ComputedMotion  SensePosition=on  SenseVelocity=off  SenseAcceleration=off  SenseTorqueForce=off  SenseLowerLimitTorqueForce=off  SenseUpperLimitTorqueForce=off  LowerLimitSpecify=off  LowerLimitBound=-80  LowerLimitBoundUnits=deg  LowerLimitStiffness=1e4  LowerLimitStiffnessUnits=N*m/deg  LowerLimitDamping=10  LowerLimitDampingUnits=N*m/(deg/s)  LowerLimitTransitionRegionWidth=0.1  LowerLimitTransitionRegionWidthUnits=deg  UpperLimitSpecify=off  UpperLimitBound=15  UpperLimitBoundUnits=deg  UpperLimitStiffness=1e4  UpperLimitStiffnessUnits=N*m/deg  UpperLimitDamping=10  UpperLimitDampingUnits=N*m/(deg/s)  UpperLimitTransitionRegionWidth=0.1  UpperLimitTransitionRegionWidthUnits=deg  PositionTargetSpecify=on  PositionTargetPriority=Low  PositionTargetValue=smiData.RevoluteJoint(4).Rz.Pos  PositionTargetValueUnits=deg  VelocityTargetSpecify=off  VelocityTargetPriority=High  VelocityTargetValue=0  VelocityTargetValueUnits=deg/s
  Rev_MR_ActAil : sm_lib/Joints/Revolute Joint  JointMode=Normal  SenseConstraintForce=off  SenseConstraintForceX=off  SenseConstraintForceY=off  SenseConstraintForceZ=off  SenseConstraintTorque=off  SenseConstraintTorqueX=off  SenseConstraintTorqueY=off  SenseConstraintTorqueZ=off  SenseTotalForce=off  SenseTotalForceX=off  SenseTotalForceY=off  SenseTotalForceZ=off  SenseTotalTorque=off  SenseTotalTorqueX=off  SenseTotalTorqueY=off  SenseTotalTorqueZ=off  CompositeWrenchDir=FollowerOnBase  CompositeWrenchFrame=BaseFrame  EquilibriumPosition=0  EquilibriumPositionUnits=rad  SpringStiffness=0  SpringStiffnessUnits=N*m/rad  DampingCoefficient=0  DampingCoefficientUnits=N*m/(rad/s)  TorqueActuationMode=NoTorque  MotionActuationMode=ComputedMotion  SensePosition=off  SenseVelocity=off  SenseAcceleration=off  SenseTorqueForce=off  SenseLowerLimitTorqueForce=off  SenseUpperLimitTorqueForce=off  LowerLimitSpecify=off  LowerLimitBound=-90  LowerLimitBoundUnits=deg  LowerLimitStiffness=1e4  LowerLimitStiffnessUnits=N*m/deg  LowerLimitDamping=10  LowerLimitDampingUnits=N*m/(deg/s)  LowerLimitTransitionRegionWidth=0.1  LowerLimitTransitionRegionWidthUnits=deg  UpperLimitSpecify=off  UpperLimitBound=90  UpperLimitBoundUnits=deg  UpperLimitStiffness=1e4  UpperLimitStiffnessUnits=N*m/deg  UpperLimitDamping=10  UpperLimitDampingUnits=N*m/(deg/s)  UpperLimitTransitionRegionWidth=0.1  UpperLimitTransitionRegionWidthUnits=deg  PositionTargetSpecify=on  PositionTargetPriority=Low  PositionTargetValue=smiData.RevoluteJoint(2).Rz.Pos  PositionTargetValueUnits=deg  VelocityTargetSpecify=off  VelocityTargetPriority=High  VelocityTargetValue=0  VelocityTargetValueUnits=deg/s
  Rev_MR_ActMount : sm_lib/Joints/Revolute Joint  JointMode=Normal  SenseConstraintForce=off  SenseConstraintForceX=off  SenseConstraintForceY=off  SenseConstraintForceZ=off  SenseConstraintTorque=off  SenseConstraintTorqueX=off  SenseConstraintTorqueY=off  SenseConstraintTorqueZ=off  SenseTotalForce=off  SenseTotalForceX=off  SenseTotalForceY=off  SenseTotalForceZ=off  SenseTotalTorque=off  SenseTotalTorqueX=off  SenseTotalTorqueY=off  SenseTotalTorqueZ=off  CompositeWrenchDir=FollowerOnBase  CompositeWrenchFrame=BaseFrame  EquilibriumPosition=0  EquilibriumPositionUnits=rad  SpringStiffness=0  SpringStiffnessUnits=N*m/rad  DampingCoefficient=0  DampingCoefficientUnits=N*m/(rad/s)  TorqueActuationMode=NoTorque  MotionActuationMode=ComputedMotion  SensePosition=on  SenseVelocity=off  SenseAcceleration=off  SenseTorqueForce=off  SenseLowerLimitTorqueForce=off  SenseUpperLimitTorqueForce=off  LowerLimitSpecify=off  LowerLimitBound=-90  LowerLimitBoundUnits=deg  LowerLimitStiffness=1e4  LowerLimitStiffnessUnits=N*m/deg  LowerLimitDamping=10  LowerLimitDampingUnits=N*m/(deg/s)  LowerLimitTransitionRegionWidth=0.1  LowerLimitTransitionRegionWidthUnits=deg  UpperLimitSpecify=off  UpperLimitBound=90  UpperLimitBoundUnits=deg  UpperLimitStiffness=1e4  UpperLimitStiffnessUnits=N*m/deg  UpperLimitDamping=10  UpperLimitDampingUnits=N*m/(deg/s)  UpperLimitTransitionRegionWidth=0.1  UpperLimitTransitionRegionWidthUnits=deg  PositionTargetSpecify=on  PositionTargetPriority=Low  PositionTargetValue=smiData.RevoluteJoint(1).Rz.Pos  PositionTargetValueUnits=deg  VelocityTargetSpecify=off  VelocityTargetPriority=High  VelocityTargetValue=0  VelocityTargetValueUnits=deg/s
  Scope : Scope  Commented=on  NumInputPorts=3
  C1 : PMIOPort  Side=Left
  P1 : PMIOPort  Port=2  Side=Left
  C2 : PMIOPort  Port=3  Side=Left
  P2 : PMIOPort  Port=4  Side=Left
  C3 : PMIOPort  Port=5  Side=Left
  P3 : PMIOPort  Port=6  Side=Left
  CG : PMIOPort  Port=7  Side=Right
  qM : Outport  VectorParamsAs1DForOutWhenUnconnected=off
  wires:
  PS-Simulink Converter/1 -> qM/1
  PS-Simulink Converter1/1 -> Scope/1
  PS-Simulink Converter2/1 -> Scope/2
  PS-Simulink Converter3/1 -> Scope/3
  connections:
  Cyl_MC_ActAil/LConn1 -- Piston2/RConn1
  Rev_MR_ActAil/LConn1 -- Piston1/RConn1
  C1/RConn1 -- Cyl1/RConn1
  Cyl2/LConn1 -- Rev_MC_ActMount/RConn1
  MountBrackets_1/RConn2 -- Rev_MR_ActMount/LConn1
  Rev_MR_ActAil/RConn1 -- Aileron_Att_1/LConn2
  Cyl_MC_ActAil/RConn1 -- Aileron_Att_1/LConn3
  MountBrackets_1/RConn3 -- Rev_MC_ActMount/LConn1
  Cyl1/LConn1 -- Rev_MR_ActMount/RConn1
  P1/RConn1 -- Piston1/LConn1
  Cyl_MC_BrkLAil/LConn1 -- MountBrackets_1/RConn1
  MountBrackets_1/RConn4 -- Rev_ML_ActMount/LConn1
  C2/RConn1 -- Cyl2/RConn1
  Aileron_Att_1/LConn1 -- Cyl_MC_BrkLAil/RConn1
  P2/RConn1 -- Piston2/LConn1
  PS-Simulink Converter/LConn1 -- Cyl_MC_BrkLAil/RConn2
  CG/RConn1 -- Aileron_Att_1/RConn1
  Rev_ML_ActMount/RConn1 -- Cyl3/LConn1
  Cyl3/RConn1 -- C3/RConn1
  Cyl_ML_ActAil/LConn1 -- Piston3/RConn1
  Aileron_Att_1/LConn4 -- Cyl_ML_ActAil/RConn1
  Piston3/LConn1 -- P3/RConn1
  PS-Simulink Converter1/LConn1 -- Rev_MR_ActMount/RConn2
  PS-Simulink Converter2/LConn1 -- Rev_MC_ActMount/RConn2
  PS-Simulink Converter3/LConn1 -- Rev_ML_ActMount/RConn2

== system GUAM/Geodetic Coordinates/M and N ==
  phi : Inport
  Constant : Constant  Value=0.081819190842622
  M and N : MATLAB Function  TreatAsAtomicUnit=on
  a : Constant  Value=6378137
  M : Outport
  N : Outport  Port=2
  wires:
  Constant/1 -> M and N/2(e)
  phi/1 -> M and N/3(phi)
  M and N/1(M) -> M/1
  a/1 -> M and N/1(a)
  M and N/2(N) -> N/1

== system GUAM/Navigational BLOCK/Navigational Equation ==
  psi : Inport
  theat : Inport  Port=2
  phi : Inport  Port=3
  Matrix Multiply : Product  Inputs=3  Multiplication=Matrix(*)
  Roationa Matrix from 2 to body : MATLAB Function  TreatAsAtomicUnit=on
  Roational Matrix from 1 to 2 : MATLAB Function  TreatAsAtomicUnit=on
  Rotaional Matrix from V to 1 : MATLAB Function  TreatAsAtomicUnit=on
  C_B/V : Outport
  wires:
  psi/1 -> Rotaional Matrix from V to 1/1(psi)
  theat/1 -> Roational Matrix from 1 to 2/1(theta)
  phi/1 -> Roationa Matrix from 2 to body/1(phi)
  Roationa Matrix from 2 to body/1(C_b_2) -> Matrix Multiply/1
  Roational Matrix from 1 to 2/1(C_2_1) -> Matrix Multiply/2
  Rotaional Matrix from V to 1/1(C_1_V) -> Matrix Multiply/3
  Matrix Multiply/1 -> C_B/V/1
